simulink model "pidcontrol_control"  (Simulink 3.00)
libraries: mathlib x4, execlib x1, reglib x1, arclib x1

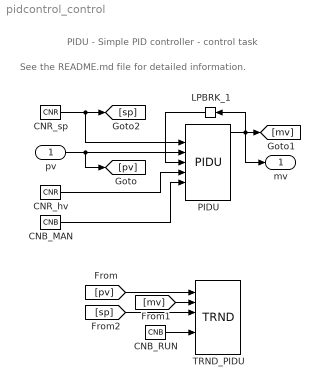
== system pidcontrol_control ==
  note: See the README.md file for detailed information.
  note: PIDU - Simple PID controller - control task
  pv : Inport  Port=1
  CNB_MAN : mathlib/CNB  YCN=off
  CNB_RUN : mathlib/CNB  YCN=on
  CNR_hv : mathlib/CNR  ycn=0
  CNR_sp : mathlib/CNR  ycn=0
  LPBRK_1 : execlib/LPBRK  Orientation=left
  PIDU : reglib/PIDU  irtype=7: PID  RACT=off  k=0.75  ti=4.3  td=1.07  nd=10  b=0.5  c=0  tt=2.1  hilim=1  lolim=-1  dz=0  icotype=1: Analog
  TRND_PIDU : arclib/TRND  n=3  l=1000  btype=8: Double  ptype1=1: Store  ptype2=1: Store  ptype3=1: Store  ptype4=1: Store  pfac=1  afac=0  arc=0  id=1  Title=Trend Title  timesrc=1
  mv : Outport  Port=1
  wires:
  CNB_MAN/1 -> PIDU/6
  CNB_RUN/1 -> TRND_PIDU/5
  CNR_hv/1 -> PIDU/5
  CNR_sp/1 -> [sp], PIDU/2
  [pv] -> TRND_PIDU/1
  [mv] -> TRND_PIDU/2
  [sp] -> TRND_PIDU/3
  LPBRK_1/1 -> PIDU/4
  PIDU/1 -> [mv], LPBRK_1/1, mv/1
  pv/1 -> [pv], PIDU/3
